simulink model "modelP21"  (R2014b)
settings: Solver=ode45  StartTime=0.0  StopTime=10.0  RelTol=1e-3
values from neighbouring files (symbols this model uses):
  Ca = [CkP19 0 0]    [mainbis.m]
  Ts = 0.0002    [mainbis.m]
undefined symbols (not defined in the file or in its folder): Fa, Ga, Gva, M
libraries: simulink x7
settings Model: Creator=titou  LastModifiedBy=titou

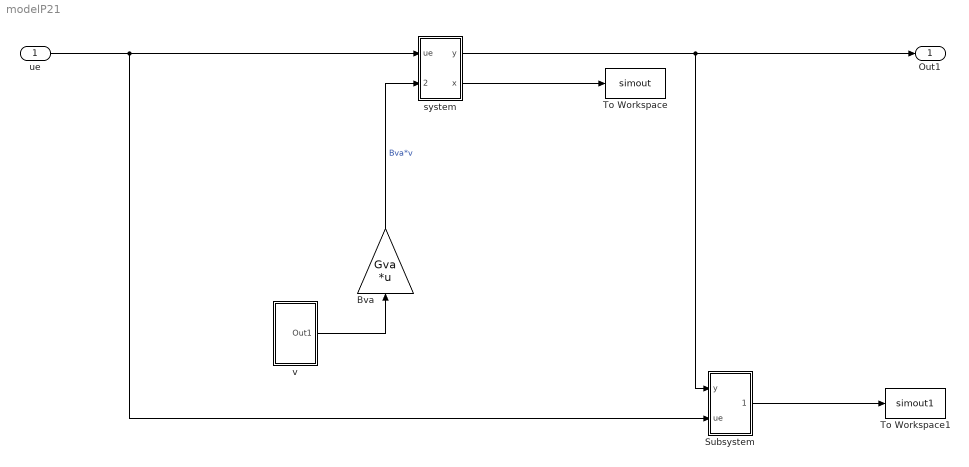
== system modelP21 ==
  ue : Inport
  Bva : Gain  Gain=Gva  Multiplication=Matrix(K*u)
  Subsystem : Subsystem
  To Workspace : ToWorkspace  VariableName=simout  SaveFormat=Timeseries  SampleTime=-1
  To Workspace1 : ToWorkspace  VariableName=simout1  SaveFormat=Timeseries  SampleTime=-1
  system : Subsystem
  v : Subsystem
  Out1 : Outport
  wires:
  ue/1 -> Subsystem/2(ue), system/1(ue)
  v/1(Out1) -> Bva/1
  system/1(y) -> Out1/1, Subsystem/1("y ")
  Bva/1 -> system/2(noise)  "Bva*v"
  system/2(x) -> To Workspace/1
  Subsystem/1(x_hat) -> To Workspace1/1

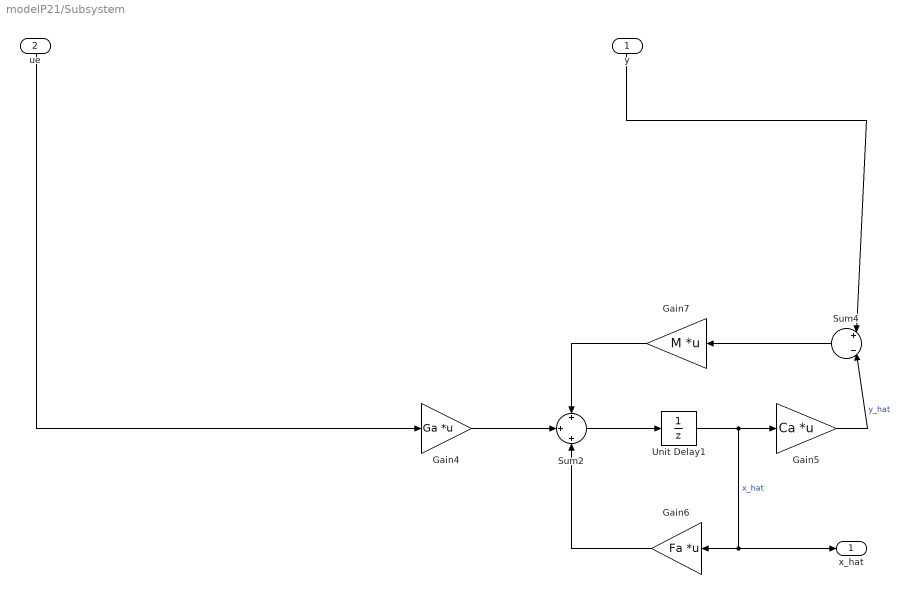
== system modelP21/Subsystem ==
  "y " : Inport
  ue : Inport  Port=2
  Gain4 : Gain  Gain=Ga  Multiplication=Matrix(K*u)
  Gain5 : Gain  Gain=Ca  Multiplication=Matrix(K*u)
  Gain6 : Gain  Gain=Fa  Multiplication=Matrix(K*u)
  Gain7 : Gain  Gain=M  Multiplication=Matrix(K*u)
  Sum2 : Sum  Inputs=+|+|+
  Sum4 : Sum  Inputs=|+|-|
  Unit Delay1 : UnitDelay  SampleTime=-1
  x_hat : Outport
  wires:
  Gain7/1 -> Sum2/1
  ue/1 -> Gain4/1
  "y "/1 -> Sum4/1
  Gain4/1 -> Sum2/2
  Unit Delay1/1 -> x_hat/1, Gain6/1, Gain5/1  "x_hat"
  Gain6/1 -> Sum2/3
  Sum2/1 -> Unit Delay1/1
  Gain5/1 -> Sum4/2  "y_hat"
  Sum4/1 -> Gain7/1

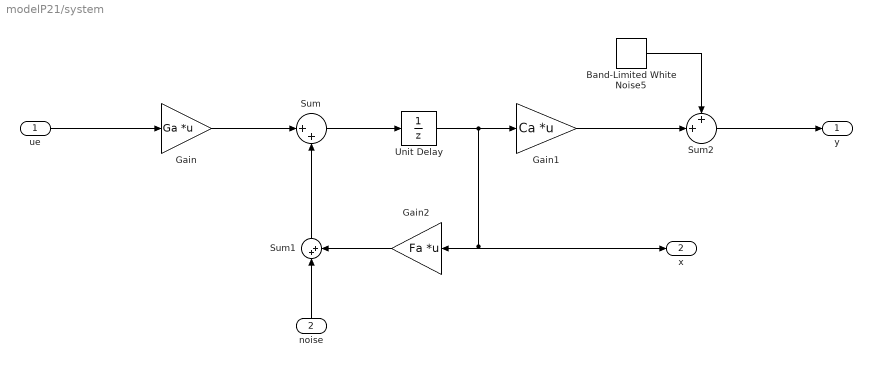
== system modelP21/system ==
  ue : Inport
  noise : Inport  Port=2
  Band-Limited White Noise5 : simulink/Sources/Band-Limited White Noise  Cov=[0.001]  Ts=Ts  seed=[193457]
  Gain : Gain  Gain=Ga  Multiplication=Matrix(K*u)
  Gain1 : Gain  Gain=Ca  Multiplication=Matrix(K*u)
  Gain2 : Gain  Gain=Fa  Multiplication=Matrix(K*u)
  Sum : Sum  Inputs=|++
  Sum1 : Sum  Inputs=|++
  Sum2 : Sum  Inputs=++|
  Unit Delay : UnitDelay  SampleTime=-1
  y : Outport
  x : Outport  Port=2
  wires:
  noise/1 -> Sum1/1
  Sum/1 -> Unit Delay/1
  Unit Delay/1 -> x/1, Gain2/1, Gain1/1
  Sum1/1 -> Sum/2
  Gain2/1 -> Sum1/2
  ue/1 -> Gain/1
  Gain/1 -> Sum/1
  Sum2/1 -> y/1
  Gain1/1 -> Sum2/2
  Band-Limited White Noise5/1 -> Sum2/1

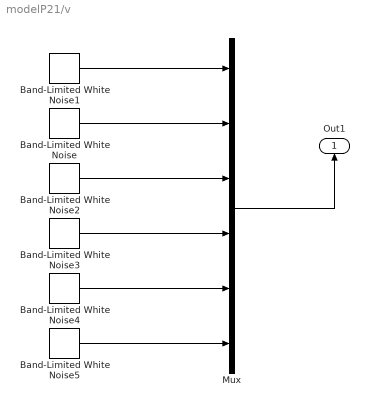
== system modelP21/v ==
  Band-Limited White Noise : simulink/Sources/Band-Limited White Noise  Cov=[0.1]  Ts=Ts  seed=[23441]
  Band-Limited White Noise1 : simulink/Sources/Band-Limited White Noise  Cov=[0.1]  Ts=Ts  seed=[123456]
  Band-Limited White Noise2 : simulink/Sources/Band-Limited White Noise  Cov=[0.1]  Ts=Ts  seed=[983245]
  Band-Limited White Noise3 : simulink/Sources/Band-Limited White Noise  Cov=[0.1]  Ts=Ts  seed=[123459]
  Band-Limited White Noise4 : simulink/Sources/Band-Limited White Noise  Cov=[0.1]  Ts=Ts  seed=[123458]
  Band-Limited White Noise5 : simulink/Sources/Band-Limited White Noise  Cov=[0.1]  Ts=Ts  seed=[123457]
  Mux : Mux  Inputs=6
  Out1 : Outport
  wires:
  Band-Limited White Noise/1 -> Mux/2
  Band-Limited White Noise4/1 -> Mux/5
  Band-Limited White Noise2/1 -> Mux/3
  Band-Limited White Noise3/1 -> Mux/4
  Band-Limited White Noise5/1 -> Mux/6
  Mux/1 -> Out1/1
  Band-Limited White Noise1/1 -> Mux/1
